simulink model "smoothUpParams"  (R2020a)
settings: Solver=FixedStepAuto  StartTime=0.0  StopTime=inf  FixedStep=0.05  RelTol=1e-3  EnableMultiTasking=on
undefined symbols (not defined in the file): Angular, Linear
libraries: robotlib x6, simulink x4
settings Model: Creator=ece446  LastModifiedBy=ivory
settings DataIOCC: ReturnWorkspaceOutputs=off
settings OptimizationCC: LifeSpan=Inf  MaxStackSize=64
settings DebuggingCC: SFUnexpectedBacktrackingDiag=warning  SFNoUnconditionalDefaultTransitionDiag=warning  ArithmeticOperatorsInVariantConditions=warning
settings HardwareCC: ProdBitPerPointer=32  ProdBitPerSizeT=32  ProdBitPerPtrDiffT=32  ProdLargestAtomicFloat=None  ProdIntDivRoundTo=Undefined  ProdEndianess=Unspecified  ProdWordSize=32  ProdHWDeviceType=Generic->Unspecified (assume 32-bit Generic)  UseEmbeddedCoderFeatures=off
settings SFSimCC: SimUseLocalCustomCode=off  CustomCodeUndefinedFunction=UseInterfaceOnly
settings RTWCC: SystemTargetFile=ert.tlc  HardwareBoard=Robot Operating System (ROS)  TLCOptions=-aInlineSetEventsForThisBaseRateFcn=TLC_FALSE -aSuppressMultiTaskScheduler=TLC_FALSE -aRateBasedStepFcn=0  TemplateMakefile=ert_default_tmf  GenerateReport=on  RTWUseLocalCustomCode=off  Toolchain=Catkin  LaunchReport=on  TargetLang=C++
settings CodeAppCC: ForceParamTrailComments=on  OperatorAnnotations=on  StateflowObjectComments=on  MATLABSourceComments=on
settings ERTTargetCC: MultiwordLength=2048  ERTCustomFileBanners=off  SupportContinuousTime=on  SupportNonInlinedSFcns=on  RemoveResetFunc=off  ModelStepFunctionPrototypeControlCompliant=off
settings ConfigComp: CovMetricSettings=dw  CovHtmlReporting=on  CovSaveCumulativeToWorkspaceVar=on  CovSaveSingleToWorkspaceVar=on  CovExternalEMLEnable=off

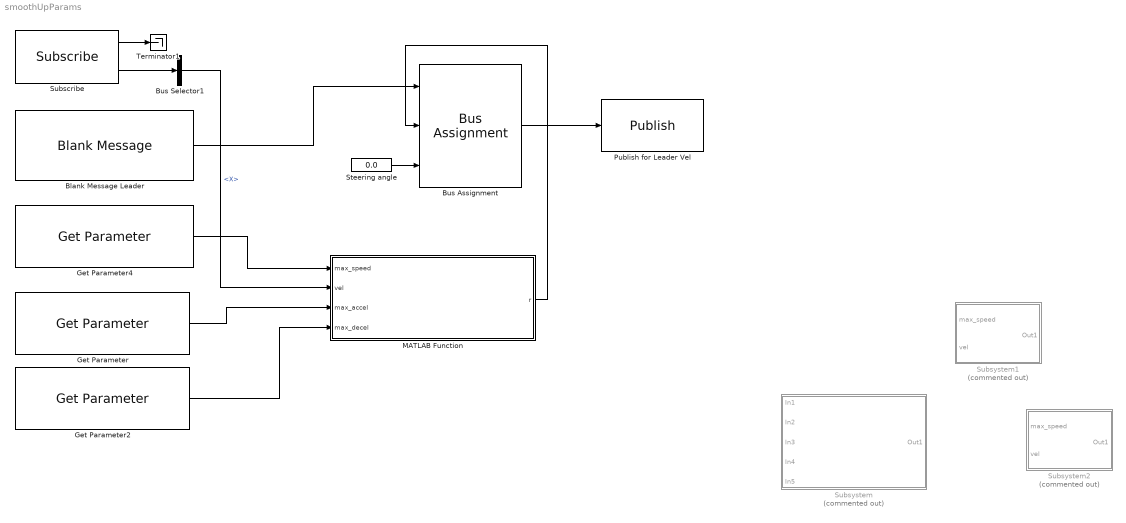
== system smoothUpParams ==
  Blank Message Leader : robotlib/Blank Message  messageClass=Message  entityType=geometry_msgs/Twist  messageType=geometry_msgs/Twist  SampleTime=inf
  Bus Assignment : BusAssignment  AssignedSignals=Linear.X,Angular.Z
  Bus Selector1 : BusSelector  OutputSignals=Linear.X
  Get Parameter : robotlib/Get Parameter  ParameterSource=Specify your own  ParameterName=max_accel  ParameterType=double  ParameterMaxArrayLength=16  ParameterInitialValue=4.5  SampleTime=-1  ShowErrorCodeOutput=off  ModelName=smoothUpParams  BlockId=ParamGet_smoothUpParams_184
      settings: SourceProductBaseCode=RR
  Get Parameter2 : robotlib/Get Parameter  ParameterSource=Specify your own  ParameterName=max_decel  ParameterType=double  ParameterMaxArrayLength=16  ParameterInitialValue=-1.5  SampleTime=-1  ShowErrorCodeOutput=off  ModelName=smoothUpParams  BlockId=ParamGet_smoothUpParams_107
      settings: SourceProductBaseCode=RR
  Get Parameter4 : robotlib/Get Parameter  ParameterSource=Specify your own  ParameterName=max_speed  ParameterType=double  ParameterMaxArrayLength=16  ParameterInitialValue=6.5  SampleTime=-1  ShowErrorCodeOutput=off  ModelName=smoothUpParams  BlockId=ParamGet_smoothUpParams_137
      settings: SourceProductBaseCode=RR
  MATLAB Function : MATLAB Function  TreatAsAtomicUnit=on
  Publish for Leader Vel : robotlib/Publish  topicSource=Specify your own  topic=cmd_vel  messageType=geometry_msgs/Twist  messageQueueLength=1
  Steering angle : Constant  Value=0.0
  Subscribe : robotlib/Subscribe  topicSource=Specify your own  topic=vel  messageType=geometry_msgs/Twist  sampleTime=-1  messageQueueLength=1
  Subsystem : Subsystem  Commented=on
  Subsystem1 : Subsystem  Commented=on
  Subsystem2 : Subsystem  Commented=on
  Terminator1 : Terminator
  wires:
  Blank Message Leader/1 -> Bus Assignment/1
  Bus Assignment/1 -> Publish for Leader Vel/1
  Steering angle/1 -> Bus Assignment/3
  Subscribe/1 -> Terminator1/1
  Subscribe/2 -> Bus Selector1/1
  Bus Selector1/1 -> MATLAB Function/2(vel)  "<X>"
  Get Parameter/1 -> MATLAB Function/3(max_accel)
  Get Parameter2/1 -> MATLAB Function/4(max_decel)
  Get Parameter4/1 -> MATLAB Function/1(max_speed)
  MATLAB Function/1(r) -> Bus Assignment/2

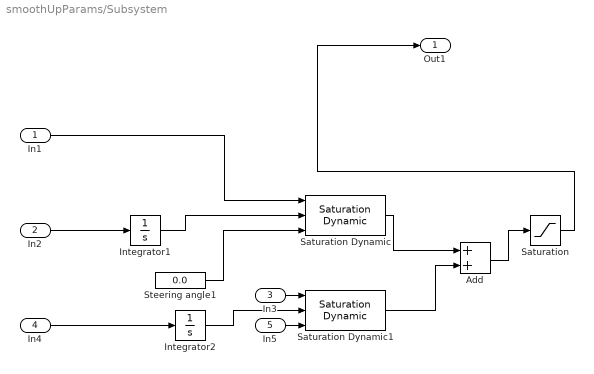
== system smoothUpParams/Subsystem ==
  In1 : Inport
  In2 : Inport  Port=2
  In3 : Inport  Port=3
  In4 : Inport  Port=4
  In5 : Inport  Port=5
  Add : Sum
  Integrator1 : Integrator
  Integrator2 : Integrator
  Saturation : Saturate  UpperLimit=inf  LowerLimit=0
  Saturation Dynamic : simulink/Discontinuities/Saturation Dynamic  OutMin=[]  OutMax=[]  OutDataTypeStr=Inherit: Same as second input  OutDataType=fixdt(1, 16)  OutScaling=2^-10  DoSatur=off
  Saturation Dynamic1 : simulink/Discontinuities/Saturation Dynamic  OutMin=[]  OutMax=[]  OutDataTypeStr=Inherit: Same as second input  OutDataType=fixdt(1, 16)  OutScaling=2^-10  DoSatur=off
  Steering angle1 : Constant  Value=0.0
  Out1 : Outport
  wires:
  In2/1 -> Integrator1/1
  Saturation Dynamic1/1 -> Add/2
  Steering angle1/1 -> Saturation Dynamic/3
  In5/1 -> Saturation Dynamic1/3
  Add/1 -> Saturation/1
  Saturation Dynamic/1 -> Add/1
  In3/1 -> Saturation Dynamic1/1
  Integrator1/1 -> Saturation Dynamic/2
  In4/1 -> Integrator2/1
  Integrator2/1 -> Saturation Dynamic1/2
  Saturation/1 -> Out1/1
  In1/1 -> Saturation Dynamic/1

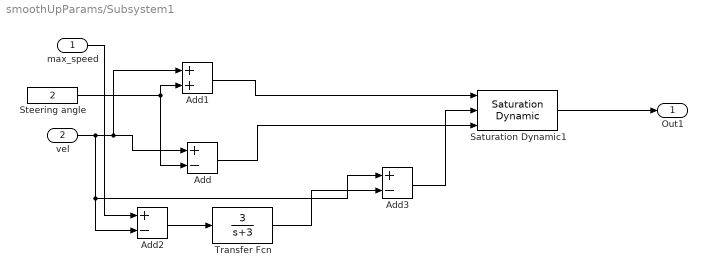
== system smoothUpParams/Subsystem1 ==
  max_speed : Inport
  vel : Inport  Port=2
  Add : Sum  Inputs=+-
  Add1 : Sum
  Add2 : Sum  Inputs=+-
  Add3 : Sum  Inputs=+-
  Saturation Dynamic1 : simulink/Discontinuities/Saturation Dynamic  OutMin=[]  OutMax=[]  OutDataTypeStr=Inherit: Same as second input  OutDataType=fixdt(1, 16)  OutScaling=2^-10  DoSatur=off
  Steering angle : Constant  Value=2
  Transfer Fcn : TransferFcn  Numerator=[3]  Denominator=[1 3]
  Out1 : Outport
  wires:
  Saturation Dynamic1/1 -> Out1/1
  vel/1 -> Add3/1, Add2/2, Add1/1, Add/1
  Steering angle/1 -> Add/2, Add1/2
  Add/1 -> Saturation Dynamic1/3
  Add1/1 -> Saturation Dynamic1/1
  max_speed/1 -> Add2/1
  Add2/1 -> Transfer Fcn/1
  Transfer Fcn/1 -> Add3/2
  Add3/1 -> Saturation Dynamic1/2

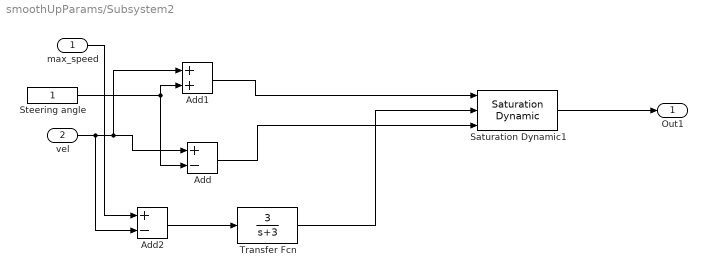
== system smoothUpParams/Subsystem2 ==
  max_speed : Inport
  vel : Inport  Port=2
  Add : Sum  Inputs=+-
  Add1 : Sum
  Add2 : Sum  Inputs=+-
  Saturation Dynamic1 : simulink/Discontinuities/Saturation Dynamic  OutMin=[]  OutMax=[]  OutDataTypeStr=Inherit: Same as second input  OutDataType=fixdt(1, 16)  OutScaling=2^-10  DoSatur=off
  Steering angle : Constant
  Transfer Fcn : TransferFcn  Numerator=[3]  Denominator=[1 3]
  Out1 : Outport
  wires:
  Saturation Dynamic1/1 -> Out1/1
  vel/1 -> Add2/2, Add1/1, Add/1
  Steering angle/1 -> Add/2, Add1/2
  Add/1 -> Saturation Dynamic1/3
  Add1/1 -> Saturation Dynamic1/1
  max_speed/1 -> Add2/1
  Add2/1 -> Transfer Fcn/1
  Transfer Fcn/1 -> Saturation Dynamic1/2

== matlab function smoothUpParams/MATLAB Function ==
  data: max_speed input; r output; vel input; max_accel input; max_decel input
function r = smoothUpParams(max_speed,vel,max_accel,max_decel)
%#codegen
% Input: max_speed = desired velocity from user
%          vel = current velocity of the vehicle
%          max_accel = maximum permissible acceleration
%         max_decel = maximum permissible deceleration
%      dx_min = minimum distance (omega_1)
% dx_activate = distance below which controller does something (omega_3)
%       decel = vector of three deceleration values for parabolas
% Out:  r =reference velocity to the Followerstopper
persistent y

if isempty(y)
    y=0;
end

% JMS: HACK timestep hacked at 0.05
dt=0.05;
if( y > max_speed + 1 )
    y = max(max_speed,y - abs(max_decel)*dt);
elseif( y < max_speed - 1)
    y = min(max_speed,y + max_accel*dt);
else
    y = double(max_speed);
end

if (y < 2 && max_speed > 2)
    y = 2;
elseif(y < 1 && max_speed > 1)
    y = 1;
end

r =min(max(y,vel-1.0),vel+2.0);
